simulink model "pendulem_cart"  (R2019b)
settings: Solver=FixedStepAuto  StartTime=0.0  StopTime=10.0  FixedStep=0.01  RelTol=1e-3
values from neighbouring files (symbols this model uses):
  d = c(4)    [EKF_estimator.m]    (also in cart_pend_EKF_script.m = 10; cart_pend_EKF_setup.m = x(8); cart_pend_HAVOK_N_train_error_sweep.m = 1; cart_pend_HAVOK_N_train_sweep.m = 1)
  g = -9.81    [EKF_estimator.m]    (also in cart_pend_EKF_script.m; cart_pend_EKF_setup.m; cart_pend_NLLS.m = 9.81; floating_pendulum_2D.m = -abs(g))
  L = c(3)    [EKF_estimator.m]    (also in cart_pend_EKF_script.m = 2; cart_pend_EKF_setup.m = x(7); cart_pend_NLLS.m = 1; floating_pendulum_2D.m = params(3))
  m = size(y_data,1)    [DMDc_param_sweep.m]    (also in EKF_estimator.m = numel(f_x); EKF_msd_estimator.m = numel(f_x); HAVOK.m = 1; HAVOK_param_sweep.m)
  M = c(2)    [EKF_estimator.m]    (also in OKID.m = 0; cart_pend_EKF_script.m = 5; cart_pend_EKF_setup.m = x(6); cart_pend_NLLS.m = 4)
settings Model: Creator=Murray  LastModifiedBy=Murray

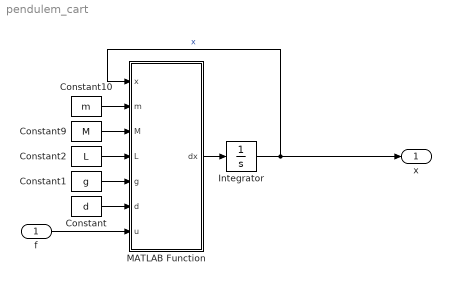
== system pendulem_cart ==
  f : Inport
  Constant : Constant  Value=d
  Constant1 : Constant  Value=g
  Constant10 : Constant  Value=m
  Constant2 : Constant  Value=L
  Constant9 : Constant  Value=M
  Integrator : Integrator  InitialCondition=[0; 0; 0; 0]
  MATLAB Function : MATLAB Function  TreatAsAtomicUnit=on
  x : Outport
  wires:
  Constant2/1 -> MATLAB Function/4(L)
  Constant9/1 -> MATLAB Function/3(M)
  Integrator/1 -> MATLAB Function/1(x), x/1  "x"
  Constant10/1 -> MATLAB Function/2(m)
  Constant1/1 -> MATLAB Function/5(g)
  MATLAB Function/1(dx) -> Integrator/1
  f/1 -> MATLAB Function/7(u)
  Constant/1 -> MATLAB Function/6(d)

== matlab function pendulem_cart/MATLAB Function ==
  data: x input; m input; M input; L input; g input; d input; u input; dx output
function dx = cartpend(x,m,M,L,g,d,u)
%CARTPEND Models a continuous system of a pendulem on a cart.
%   based on Steve Brunton code. See youtube.com/watch?v=qjhAAQexzLg&list=PLMrJAkhIeNNR20Mz-VpzgfQs5zrYi085m&index=12
%   x  = state vector [x; x_dot; theta; theta_dot]
%   dx = derivative of state vector
%   u  = input vector [f]
%   m  = mass of pendulem end
%   M  = mass of cart
%   L  = length of pendulem rod
%   g  = acceleration due to gravity
%   d  = damping coef of friction on cart

Sx = sin(x(3));
Cx = cos(x(3));
D = m*L*L*(M+m*(1-Cx^2));

dx = zeros(4,1);

dx(1,1) = x(2);
dx(2,1) = (1/D)*(-m^2*L^2*g*Cx*Sx + m*L^2*(m*L*x(4)^2*Sx - d*x(2))) + m*L*L*(1/D)*u;
dx(3,1) = x(4);
dx(4,1) = (1/D)*((m+M)*m*g*L*Sx - m*L*Cx*(m*L*x(4)^2*Sx - d*x(2))) - m*L*Cx*(1/D)*u; % +.01*randn;
